simulink model "WZhShPID2"  (Simulink 5.0)
settings: Solver=ode4  SolverMode=SingleTasking  StartTime=0.0  StopTime=1  FixedStep=0.001  RelTol=1e-3
settings Model: LastModifiedBy=ThinkPad

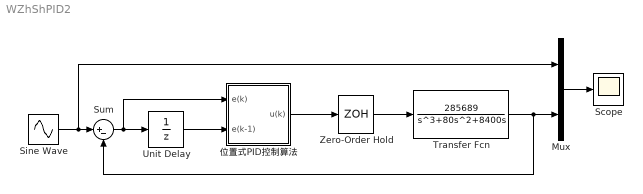
== system WZhShPID2 ==
  Mux : Mux  Inputs=2
  Scope : Scope
      settings: YMin=0  YMax=1.4  SaveName=WZhShPID2  DataFormat=Array  MaxDataPoints=50000
  Sine Wave : Sin  Amplitude=0.5  Frequency=4*pi  SampleTime=0
  Sum : Sum  Inputs=|+-  SaturateOnIntegerOverflow=on
  Transfer Fcn : TransferFcn  Numerator=[285689]  Denominator=[1 80 8400 0]
  Unit Delay : UnitDelay  SampleTime=0.001
  Zero-Order Hold : ZeroOrderHold  SampleTime=0.001
  "位置式PID控制算法 " : Subsystem
  wires:
  Sine Wave/1 -> Sum/1, Mux/1
  Sum/1 -> "位置式PID控制算法 "/1(e(k)), Unit Delay/1
  Mux/1 -> Scope/1
  Transfer Fcn/1 -> Sum/2, Mux/2
  Unit Delay/1 -> "位置式PID控制算法 "/2(e(k-1))
  "位置式PID控制算法 "/1(u(k)) -> Zero-Order Hold/1
  Zero-Order Hold/1 -> Transfer Fcn/1

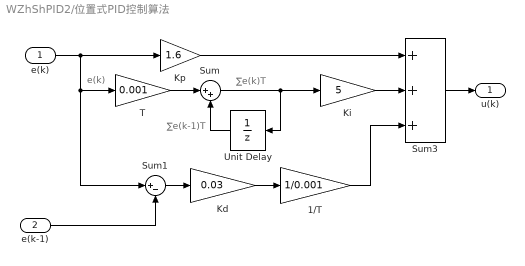
== system WZhShPID2/位置式PID控制算法  ==
  note: e(k)
  note: ∑e(k)T
  note: ∑e(k-1)T
  e(k) : Inport
  e(k-1) : Inport  Port=2
  1/T : Gain  Gain=1/0.001  SaturateOnIntegerOverflow=on
  Kd : Gain  Gain=0.03  SaturateOnIntegerOverflow=on
  Ki : Gain  Gain=5  SaturateOnIntegerOverflow=on
  Kp : Gain  Gain=1.6  SaturateOnIntegerOverflow=on
  Sum : Sum  Inputs=|++  SaturateOnIntegerOverflow=on
  Sum1 : Sum  Inputs=|+-  SaturateOnIntegerOverflow=on
  Sum3 : Sum  Inputs=+++  SaturateOnIntegerOverflow=on
  T : Gain  Gain=0.001  SaturateOnIntegerOverflow=on
  Unit Delay : UnitDelay  Orientation=left  SampleTime=0.001
  u(k) : Outport
  wires:
  Sum1/1 -> Kd/1
  e(k)/1 -> Kp/1, Sum1/1, T/1
  Kp/1 -> Sum3/1
  Ki/1 -> Sum3/2
  Sum3/1 -> u(k)/1
  Kd/1 -> 1/T/1
  1/T/1 -> Sum3/3
  Sum/1 -> Unit Delay/1, Ki/1
  Unit Delay/1 -> Sum/2
  e(k-1)/1 -> Sum1/2
  T/1 -> Sum/1
